simulink model "SPWM_Inverters"  (R2023a)
settings: Solver=ode23tb  StartTime=0.0  StopTime=1  MaxStep=1e-4  RelTol=1e-3
libraries: spsMosfetLib x22, spsSeriesRLCBranchLib x11, simulink x9, spsThreePhaseSeriesRLCBranchLib x8, spsDCVoltageSourceLib x7, spsVoltageMeasurementLib x7, spsThreePhaseVIMeasurementLib x6, spsGroundLib x3, spsPWMGenerator2LevelLib x2, spsUniversalBridgeLib x2, slpidlib x1, spsRMSLib x1
settings Model: Creator=gaming3  LastModifiedBy=gaming3

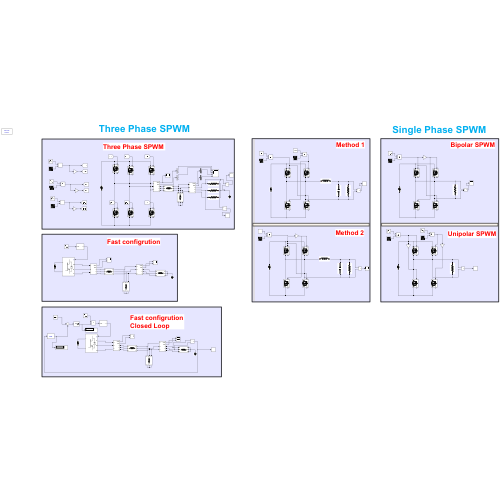
[thumbnail: Simulink's stored preview of the top-level diagram]
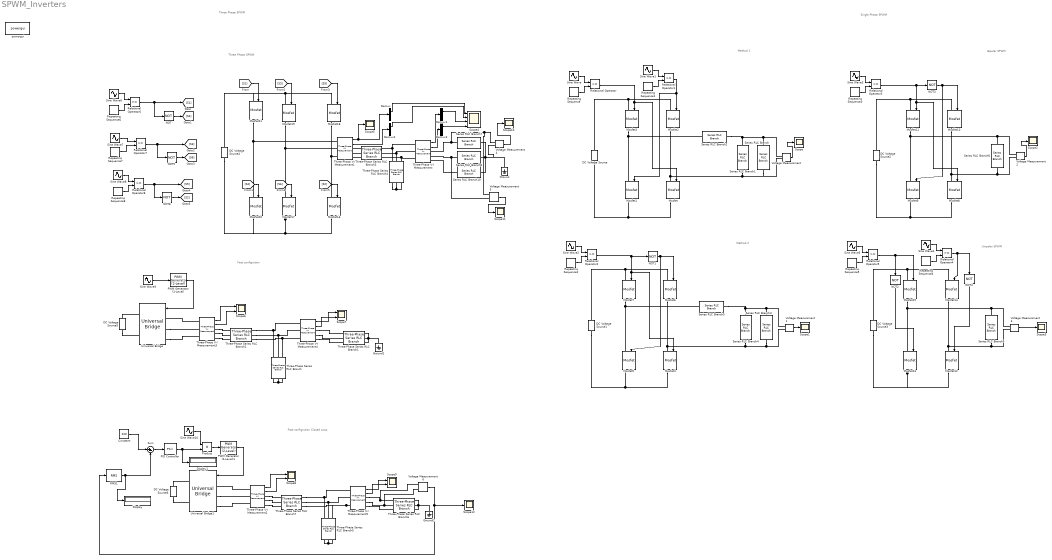
== system SPWM_Inverters ==
  note: Fast configrution
  note: Three Phase SPWM
  note: Bipolar SPWM
  note: Single Phase SPWM
  note: Unipolar SPWM
  note: Method 1
  note: Method 2
  note: Three Phase SPWM
  note: Fast configrution Closed Loop
  Constant : Constant  Value=220
  DC Voltage Source{,1..6} (7 alike) : spsDCVoltageSourceLib/DC Voltage Source  Amplitude=310  Measurements=None
  Demux{,1..3} (4 alike) : Demux  Outputs=3
  Display : Display
  Display1 : Display
  Ground : spsGroundLib/Ground  LConnTagsString=a
  Ground1 : spsGroundLib/Ground  LConnTagsString=a
  Ground2 : spsGroundLib/Ground  LConnTagsString=a
  Mosfet{,1..21} (22 alike) : spsMosfetLib/Mosfet  Ron=0.1  Lon=0  Rd=0.01  Vfd=0  IC=0  Rs=1e5  Cs=inf  Measurements=on
  NOT{,1..6} (7 alike) : Logic  Operator=NOT  IconShape=distinctive  AllPortsSameDT=off  OutDataTypeStr=boolean
  PID Controller : slpidlib/PID Controller  Controller=PI  Form=Parallel  TimeDomain=Continuous-time  UseExternalTs=off  SampleTime=-1  IntegratorMethod=Forward Euler  FilterMethod=Forward Euler  ControllerParametersSource=internal  P=0.0001  I=0.1  UseKiTs=off  D=0  N=100  UseFilter=on  TunerSelectOption=Transfer Function Based (PID Tuner App)  InitialConditionSource=internal  InitialConditionForIntegrator=0  InitialConditionForFilter=0  DifferentiatorICPrevScaledInput=0  ExternalReset=none  TrackingMode=off  Kt=1  LimitOutput=on  SatLimitsSource=internal  UpperSaturationLimit=0.98  LowerSaturationLimit=0  LinearizeAsGain=on  AntiWindupMode=none  Kb=1  LimitIntegrator=off  UpperIntegratorSaturationLimit=inf  LowerIntegratorSaturationLimit=-inf  POutMin=[]  POutMax=[]  IOutMin=[]  IOutMax=[]  DOutMin=[]  DOutMax=[]  NOutMin=[]  NOutMax=[]  SumOutMin=[]  SumOutMax=[]  SaturationOutMin=[]  SaturationOutMax=[]  PParamMin=[]  PParamMax=[]  IParamMin=[]  IParamMax=[]  DParamMin=[]  DParamMax=[]  NParamMin=[]  NParamMax=[]  KbParamMin=[]  KbParamMax=[]  KtParamMin=[]  KtParamMax=[]  KbOutMin=[]  KbOutMax=[]  KtOutMin=[]  KtOutMax=[]  IntegratorOutMin=[]  IntegratorOutMax=[]  FilterOutMin=[]  FilterOutMax=[]  SumI1OutMin=[]  SumI1OutMax=[]  SumI2OutMin=[]  SumI2OutMax=[]  SumI3OutMin=[]  SumI3OutMax=[]  SumI4OutMin=[]  SumI4OutMax=[]  SumDOutMin=[]  SumDOutMax=[]  DifferentiatorOutMin=[]  DifferentiatorOutMax=[]  FilterDiffOutCoefMin=[]  FilterDiffOutCoefMax=[]  ReciprocalOutMin=[]  ReciprocalOutMax=[]  SumDenOutMin=[]  SumDenOutMax=[]  SumNumOutMin=[]  SumNumOutMax=[]  DivideOutMin=[]  DivideOutMax=[]  UdiffTsProdOutMin=[]  UdiffTsProdOutMax=[]  NTsProdOutMin=[]  NTsProdOutMax=[]  UintegralTsProdOutMin=[]  UintegralTsProdOutMax=[]  UngainTsProdOutMin=[]  UngainTsProdOutMax=[]  ClampingZeroOutDataTypeStr=Inherit: Inherit via back propagation  ClampingZeroOutMin=[]  ClampingZeroOutMax=[]  FilterDenConstantOutDataTypeStr=Inherit: Inherit via back propagation  FilterDenConstantOutMin=[]  FilterDenConstantOutMax=[]  PCopyOutDataTypeStr=Inherit: Inherit via back propagation  PCopyOutMin=[]  PCopyOutMax=[]  NCopyOutDataTypeStr=Inherit: Inherit via back propagation  NCopyOutMin=[]  NCopyOutMax=[]  IntegratorContinuousStateAttributes=''  IntegratorStateMustResolveToSignalObject=off  IntegratorRTWStateStorageClass=Auto  FilterContinuousStateAttributes=''  FilterStateMustResolveToSignalObject=off  FilterRTWStateStorageClass=Auto  ParallelPVariant=InternalParameters  IdealPVariant=Disabled  IVariant=InternalParameters  DVariant=Disabled  IntegratorVariant=Continuous  SatVariant=Enabled  AWVariant=Passthrough  PCopyVariant=Disabled  TRVariant=Disabled  FdbkBlocksVariant=Forward  IdealPFdbkVariant=Disabled  SatFdbkVariant=Disabled  DerivativeFilterVariant=Disabled  NVariant=Disabled  NCopyVariant=Disabled_SignalSpec  FilterICVariant=Disabled  IntegratorICVariant=InternalICs  ExternalResetVariant=Disabled  TRSumVariant=Passthrough  SumFdbkVariant=Disabled  SumVariant=Sum_PI  TsampFilterVariant=InternalTs  TsampNgainVariant=Passthrough  TsampIntegralVariant=Disabled_SignalSpec  ExternalSaturationOutDataTypeStr=Inherit: Same as second input
  PWM Generator (2-Level) : spsPWMGenerator2LevelLib/PWM Generator (2-Level)  ModulatorType=Three-phase bridge (6 pulses)  ModulatorMode=Unsynchronized  Fc=101*50  Pc=90  nF=27  MinMax="[ -1  1 ]"  SamplingTechnique=Natural  ModulatingSignals=off  m=0.8  Freq=60  Phase=0  Ts=0  ShowCarrierOutport=off
  PWM Generator (2-Level)1 : spsPWMGenerator2LevelLib/PWM Generator (2-Level)  ModulatorType=Three-phase bridge (6 pulses)  ModulatorMode=Unsynchronized  Fc=101*50  Pc=90  nF=27  MinMax="[ -1  1 ]"  SamplingTechnique=Natural  ModulatingSignals=off  m=0.8  Freq=60  Phase=0  Ts=0  ShowCarrierOutport=off
  Product : Product
  RMS1 : spsRMSLib/RMS  TrueRMS=on  Freq=50  RMSInit=0  Ts=0
  Relational Operator{,1..8} (9 alike) : RelationalOperator  OutDataTypeStr=boolean  RndMeth=Simplest  InputSameDT=off
  Repeating Sequence{,1..5} (6 alike) : simulink/Sources/Repeating Sequence  rep_seq_t=[0 (1/5000)/4 (1/5000)/2 (3/5000)/4 (1/5000)]  rep_seq_y=[0 1 0 -1 0]
  Repeating Sequence6 : simulink/Sources/Repeating Sequence  rep_seq_t=[0 (0.25/5000) (0.5/5000) (0.75/5000) (1/5000)]  rep_seq_y=[0 1 0 -1 0]
  Repeating Sequence7 : simulink/Sources/Repeating Sequence  rep_seq_t=[0 (0.25/5000) (0.5/5000) (0.75/5000) (1/5000)]  rep_seq_y=[0 1 0 -1 0]
  Repeating Sequence8 : simulink/Sources/Repeating Sequence  rep_seq_t=[0 (0.25/5000) (0.5/5000) (0.75/5000) (1/5000)]  rep_seq_y=[0 1 0 -1 0]
  Scope{,1..3,5,10..12} (8 alike) : Scope
  Scope4 : Scope  NumInputPorts=4
  Scope{6..9} (4 alike) : Scope  NumInputPorts=2
  Series RLC Branch{,3,6,9} (4 alike) : spsSeriesRLCBranchLib/Series RLC Branch  LConnTagsString=__new0  RConnTagsString=__new0  BranchType=R  Resistance=100  Inductance=1e-3  SetiL0=off  InitialCurrent=0  Capacitance=1e-6  Setx0=off  InitialVoltage=0  Measurements=None
  Series RLC Branch1 : spsSeriesRLCBranchLib/Series RLC Branch  LConnTagsString=__new0  RConnTagsString=__new0  BranchType=C  Resistance=100  Inductance=1e-3  SetiL0=off  InitialCurrent=0  Capacitance=1000e-6  Setx0=off  InitialVoltage=0  Measurements=None
  Series RLC Branch10 : spsSeriesRLCBranchLib/Series RLC Branch  LConnTagsString=__new0  RConnTagsString=__new0  BranchType=R  Resistance=10  Inductance=1e-3  SetiL0=off  InitialCurrent=0  Capacitance=1e-6  Setx0=off  InitialVoltage=0  Measurements=None
  Series RLC Branch2 : spsSeriesRLCBranchLib/Series RLC Branch  LConnTagsString=__new0  RConnTagsString=__new0  BranchType=L  Resistance=100  Inductance=0.00001  SetiL0=off  InitialCurrent=0  Capacitance=1e-6  Setx0=off  InitialVoltage=0  Measurements=None
  Series RLC Branch4 : spsSeriesRLCBranchLib/Series RLC Branch  LConnTagsString=__new0  RConnTagsString=__new0  BranchType=C  Resistance=100  Inductance=1e-3  SetiL0=off  InitialCurrent=0  Capacitance=500e-6  Setx0=off  InitialVoltage=0  Measurements=None
  Series RLC Branch5 : spsSeriesRLCBranchLib/Series RLC Branch  LConnTagsString=__new0  RConnTagsString=__new0  BranchType=L  Resistance=100  Inductance=0.001  SetiL0=off  InitialCurrent=0  Capacitance=1e-6  Setx0=off  InitialVoltage=0  Measurements=None
  Series RLC Branch7 : spsSeriesRLCBranchLib/Series RLC Branch  LConnTagsString=__new0  RConnTagsString=__new0  BranchType=R  Resistance=10  Inductance=1e-3  SetiL0=off  InitialCurrent=0  Capacitance=1e-6  Setx0=off  InitialVoltage=0  Measurements=None
  Series RLC Branch8 : spsSeriesRLCBranchLib/Series RLC Branch  LConnTagsString=__new0  RConnTagsString=__new0  BranchType=R  Resistance=10  Inductance=1e-3  SetiL0=off  InitialCurrent=0  Capacitance=1e-6  Setx0=off  InitialVoltage=0  Measurements=None
  Sine Wave{,2..3,5} (4 alike) : Sin  Amplitude=0.95  Frequency=100*pi  SampleTime=0
  Sine Wave1 : Sin  Amplitude=0.95  Frequency=100*pi  Phase=pi  SampleTime=0
  Sine Wave10 : Sin  Frequency=100*pi  Phase="[0 -(2*pi)/3  (2*pi)/3 ]"  SampleTime=0
  Sine Wave4 : Sin  Amplitude=0.95  Frequency=100*pi  Phase=pi  SampleTime=0
  Sine Wave6 : Sin  Amplitude=.99  Frequency=100*pi  SampleTime=0
  Sine Wave7 : Sin  Amplitude=0.99  Frequency=100*pi  Phase=(2*pi)/3  SampleTime=0
  Sine Wave8 : Sin  Amplitude=0.99  Frequency=100*pi  Phase=(4*pi)/3  SampleTime=0
  Sine Wave9 : Sin  Amplitude=0.99  Frequency=100*pi  Phase="[0 -(2*pi)/3  (2*pi)/3 ]"  SampleTime=0
  Sum : Sum  Inputs=|+-
  Three-Phase Series RLC Branch : spsThreePhaseSeriesRLCBranchLib/Three-Phase Series RLC Branch  LConnTagsString=A|B|C  RConnTagsString=A|B|C  BranchType=C  Resistance=1  Inductance=1e-3  Capacitance=500e-6  Measurements=None
  Three-Phase Series RLC Branch1 : spsThreePhaseSeriesRLCBranchLib/Three-Phase Series RLC Branch  LConnTagsString=A|B|C  RConnTagsString=A|B|C  BranchType=R  Resistance=10  Inductance=1e-3  Capacitance=1e-6  Measurements=None
  Three-Phase Series RLC Branch2 : spsThreePhaseSeriesRLCBranchLib/Three-Phase Series RLC Branch  LConnTagsString=A|B|C  RConnTagsString=A|B|C  BranchType=L  Resistance=1  Inductance=5e-3  Capacitance=1e-6  Measurements=None
  Three-Phase Series RLC Branch3 : spsThreePhaseSeriesRLCBranchLib/Three-Phase Series RLC Branch  LConnTagsString=A|B|C  RConnTagsString=A|B|C  BranchType=L  Resistance=1  Inductance=5e-3  Capacitance=1e-6  Measurements=None
  Three-Phase Series RLC Branch4 : spsThreePhaseSeriesRLCBranchLib/Three-Phase Series RLC Branch  LConnTagsString=A|B|C  RConnTagsString=A|B|C  BranchType=C  Resistance=1  Inductance=1e-3  Capacitance=500e-6  Measurements=None
  Three-Phase Series RLC Branch5 : spsThreePhaseSeriesRLCBranchLib/Three-Phase Series RLC Branch  LConnTagsString=A|B|C  RConnTagsString=A|B|C  BranchType=C  Resistance=1  Inductance=1e-3  Capacitance=500e-6  Measurements=None
  Three-Phase Series RLC Branch6 : spsThreePhaseSeriesRLCBranchLib/Three-Phase Series RLC Branch  LConnTagsString=A|B|C  RConnTagsString=A|B|C  BranchType=R  Resistance=10  Inductance=1e-3  Capacitance=1e-6  Measurements=None
  Three-Phase Series RLC Branch7 : spsThreePhaseSeriesRLCBranchLib/Three-Phase Series RLC Branch  LConnTagsString=A|B|C  RConnTagsString=A|B|C  BranchType=L  Resistance=1  Inductance=5e-3  Capacitance=1e-6  Measurements=None
  Three-Phase V-I Measurement : spsThreePhaseVIMeasurementLib/Three-Phase V-I Measurement  VoltageMeasurement=phase-to-phase  SetLabelV=off  LabelV=Vabc  Vpu=off  VpuLL=off  CurrentMeasurement=yes  SetLabelI=off  LabelI=Iabc  Ipu=off  Pbase=100e6  Vbase=500e3  OutputType=Complex  PhasorSimulation=off  PSBequivalent=0
  Three-Phase V-I Measurement1 : spsThreePhaseVIMeasurementLib/Three-Phase V-I Measurement  VoltageMeasurement=phase-to-ground  SetLabelV=off  LabelV=Vabc  Vpu=off  VpuLL=off  CurrentMeasurement=yes  SetLabelI=off  LabelI=Iabc  Ipu=off  Pbase=100e6  Vbase=500e3  OutputType=Complex  PhasorSimulation=off  PSBequivalent=0
  Three-Phase V-I Measurement2 : spsThreePhaseVIMeasurementLib/Three-Phase V-I Measurement  VoltageMeasurement=phase-to-phase  SetLabelV=off  LabelV=Vabc  Vpu=off  VpuLL=off  CurrentMeasurement=yes  SetLabelI=off  LabelI=Iabc  Ipu=off  Pbase=100e6  Vbase=500e3  OutputType=Complex  PhasorSimulation=off  PSBequivalent=0
  Three-Phase V-I Measurement3 : spsThreePhaseVIMeasurementLib/Three-Phase V-I Measurement  VoltageMeasurement=phase-to-phase  SetLabelV=off  LabelV=Vabc  Vpu=off  VpuLL=off  CurrentMeasurement=yes  SetLabelI=off  LabelI=Iabc  Ipu=off  Pbase=100e6  Vbase=500e3  OutputType=Complex  PhasorSimulation=off  PSBequivalent=0
  Three-Phase V-I Measurement4 : spsThreePhaseVIMeasurementLib/Three-Phase V-I Measurement  VoltageMeasurement=phase-to-ground  SetLabelV=off  LabelV=Vabc  Vpu=off  VpuLL=off  CurrentMeasurement=yes  SetLabelI=off  LabelI=Iabc  Ipu=off  Pbase=100e6  Vbase=500e3  OutputType=Complex  PhasorSimulation=off  PSBequivalent=0
  Three-Phase V-I Measurement5 : spsThreePhaseVIMeasurementLib/Three-Phase V-I Measurement  VoltageMeasurement=phase-to-ground  SetLabelV=off  LabelV=Vabc  Vpu=off  VpuLL=off  CurrentMeasurement=yes  SetLabelI=off  LabelI=Iabc  Ipu=off  Pbase=100e6  Vbase=500e3  OutputType=Complex  PhasorSimulation=off  PSBequivalent=0
  Universal Bridge : spsUniversalBridgeLib/Universal Bridge  Arms=3  SnubberResistance=1e5  SnubberCapacitance=inf  Device=IGBT / Diodes  Ron=1e-3  Lon=0  ForwardVoltages="[  0  0  ]"  ForwardVoltage=0  GTOparameters=[ 10e-6 , 20e-6 ]  IGBTparameters=[ 1e-6 , 2e-6 ]  Measurements=None  Measurements_2=None  converterType=Rectifier
  Universal Bridge1 : spsUniversalBridgeLib/Universal Bridge  Arms=3  SnubberResistance=1e5  SnubberCapacitance=inf  Device=IGBT / Diodes  Ron=1e-3  Lon=0  ForwardVoltages="[  0  0  ]"  ForwardVoltage=0  GTOparameters=[ 10e-6 , 20e-6 ]  IGBTparameters=[ 1e-6 , 2e-6 ]  Measurements=None  Measurements_2=None  converterType=Rectifier
  Voltage Measurement{,1..6} (7 alike) : spsVoltageMeasurementLib/Voltage Measurement  PhasorSimulation=off  OutputType=Complex  PSBequivalent=0
  powergui : spspowerguiLib/powergui  Priority=1  SimulationMode=Discrete  SampleTime=1e-06  frequency=60  Iterations=50  frequencyindice=0  Pbase=100e6  ErrMax=1e-4  UnitsV=kV  UnitsW=MW  buscounter=0  FunctionMessages=off  echomessages=off  EnableUseOfTLC=off  CurrentSourceSwitches=off  DisableSnubberDevices=off  DisableRonSwitches=off  DisableVfSwitches=off  DisplayEquations=off  AutomaticDiscreteSolvers=off  SolverType=Tustin/Backward Euler (TBE)  Interpol=off  ExternalGateDelay=off  methode=off  Ts=100  x0status=blocks  SPID=on  SwTol=0  HookPort=off  NonlinearTolerance=1e-4  nMaxIteration=100  ContinueOnMaxIteration=off  RestoreLinks=warning  ResistiveCurrentMeasurement=off  Frange=[0:2:500]  Ylog=off  Xlog=on  ShowGrid=off  save=off  variable=ZData  structure=0  ZoomFFT=off  StartTime=0.0  cycles=1  DisplayStyle=1  fundamental=60  FreqAxis=off  MaxFrequency=1000  frequencyindicesteady=1  RmsSteady=1  display=off
  wires:
  Voltage Measurement/1 -> Scope/1
  Sine Wave/1 -> Relational Operator/1
  Repeating Sequence/1 -> Relational Operator/2
  Relational Operator/1 -> Mosfet/1, Mosfet3/1
  Repeating Sequence1/1 -> Relational Operator1/2
  Sine Wave1/1 -> Relational Operator1/1
  Relational Operator1/1 -> Mosfet1/1, Mosfet2/1
  Relational Operator2/1 -> NOT1/1, Mosfet7/1, Mosfet4/1
  Repeating Sequence2/1 -> Relational Operator2/2
  Sine Wave2/1 -> Relational Operator2/1
  Voltage Measurement1/1 -> Scope1/1
  NOT1/1 -> Mosfet6/1, Mosfet5/1
  Voltage Measurement3/1 -> Scope3/1
  Sine Wave5/1 -> Relational Operator5/1
  Repeating Sequence5/1 -> Relational Operator5/2
  Relational Operator5/1 -> Mosfet15/1, NOT2/1
  Relational Operator3/1 -> NOT3/1, Mosfet11/1, Mosfet8/1
  Repeating Sequence3/1 -> Relational Operator3/2
  Sine Wave3/1 -> Relational Operator3/1
  Voltage Measurement2/1 -> Scope2/1
  NOT3/1 -> Mosfet10/1, Mosfet9/1
  NOT2/1 -> Mosfet13/1
  Relational Operator4/1 -> NOT4/1, Mosfet14/1
  Repeating Sequence4/1 -> Relational Operator4/2
  Sine Wave4/1 -> Relational Operator4/1
  NOT4/1 -> Mosfet12/1
  [S6] -> Mosfet17/1
  NOT6/1 -> [S2]
  Three-Phase V-I Measurement/1 -> Demux1/1
  [S5] -> Mosfet18/1
  Three-Phase V-I Measurement1/1 -> Demux/1, Scope5/1
  [S1] -> Mosfet21/1
  Demux1/1 -> Scope4/3
  Demux/1 -> Scope4/1
  [S4] -> Mosfet20/1
  Demux3/1 -> Scope4/4
  Relational Operator7/1 -> [S3], NOT5/1
  Demux2/1 -> Scope4/2
  NOT5/1 -> [S6]
  NOT/1 -> [S4]
  Three-Phase V-I Measurement1/2 -> Demux2/1
  [S3] -> Mosfet19/1
  [S2] -> Mosfet16/1
  Three-Phase V-I Measurement/2 -> Demux3/1
  Repeating Sequence6/1 -> Relational Operator6/2
  Sine Wave6/1 -> Relational Operator6/1
  Relational Operator6/1 -> NOT/1, [S1]
  Repeating Sequence7/1 -> Relational Operator7/2
  Sine Wave8/1 -> Relational Operator8/1
  Repeating Sequence8/1 -> Relational Operator8/2
  Relational Operator8/1 -> NOT6/1, [S5]
  Sine Wave7/1 -> Relational Operator7/1
  Sine Wave9/1 -> PWM Generator (2-Level)/1
  PWM Generator (2-Level)/1 -> Universal Bridge/1
  Three-Phase V-I Measurement3/1 -> Scope6/1
  Three-Phase V-I Measurement3/2 -> Scope6/2
  Three-Phase V-I Measurement4/1 -> Scope7/1
  Three-Phase V-I Measurement4/2 -> Scope7/2
  Three-Phase V-I Measurement5/2 -> Scope9/2
  Three-Phase V-I Measurement5/1 -> Scope9/1
  Three-Phase V-I Measurement2/2 -> Scope8/2
  Three-Phase V-I Measurement2/1 -> Scope8/1
  PWM Generator (2-Level)1/1 -> Universal Bridge1/1
  Voltage Measurement4/1 -> Scope10/1
  Voltage Measurement5/1 -> Scope11/1
  Product/1 -> PWM Generator (2-Level)1/1
  Sine Wave10/1 -> Product/1
  RMS1/1 -> Display/1, Sum/2
  Constant/1 -> Sum/1
  Sum/1 -> PID Controller/1
  PID Controller/1 -> Display1/1, Product/2
  Voltage Measurement6/1 -> Scope12/1, RMS1/1
  connections:
  Mosfet3/LConn1 -- DC Voltage Source/RConn1 -- Mosfet2/LConn1
  Voltage Measurement/LConn1 -- Series RLC Branch/LConn1 -- Series RLC Branch1/LConn1 -- Series RLC Branch2/RConn1
  Mosfet2/RConn1 -- Series RLC Branch/RConn1 -- Voltage Measurement/LConn2 -- Series RLC Branch1/RConn1 -- Mosfet/LConn1
  Mosfet/RConn1 -- DC Voltage Source/LConn1 -- Mosfet1/RConn1
  Mosfet3/RConn1 -- Series RLC Branch2/LConn1 -- Mosfet1/LConn1
  DC Voltage Source1/RConn1 -- Mosfet7/LConn1 -- Mosfet6/LConn1
  Series RLC Branch3/LConn1 -- Voltage Measurement1/LConn1 -- Series RLC Branch5/RConn1 -- Series RLC Branch4/LConn1
  Series RLC Branch3/RConn1 -- Voltage Measurement1/LConn2 -- Series RLC Branch4/RConn1 -- Mosfet4/LConn1 -- Mosfet6/RConn1
  Mosfet4/RConn1 -- Mosfet5/RConn1 -- DC Voltage Source1/LConn1
  Series RLC Branch5/LConn1 -- Mosfet7/RConn1 -- Mosfet5/LConn1
  DC Voltage Source2/RConn1 -- Mosfet11/LConn1 -- Mosfet10/LConn1
  Series RLC Branch6/RConn1 -- Voltage Measurement2/LConn2 -- Mosfet8/LConn1 -- Mosfet10/RConn1
  Mosfet8/RConn1 -- Mosfet9/RConn1 -- DC Voltage Source2/LConn1
  Series RLC Branch6/LConn1 -- Mosfet9/LConn1 -- Mosfet11/RConn1 -- Voltage Measurement2/LConn1
  Mosfet15/LConn1 -- DC Voltage Source3/RConn1 -- Mosfet14/LConn1
  Voltage Measurement3/LConn2 -- Mosfet14/RConn1 -- Mosfet12/LConn1 -- Series RLC Branch9/RConn1
  Mosfet13/RConn1 -- Mosfet12/RConn1 -- DC Voltage Source3/LConn1
  Voltage Measurement3/LConn1 -- Mosfet15/RConn1 -- Mosfet13/LConn1 -- Series RLC Branch9/LConn1
  Mosfet19/RConn1 -- Three-Phase V-I Measurement1/LConn2 -- Mosfet17/LConn1
  Mosfet19/LConn1 -- DC Voltage Source4/RConn1 -- Mosfet21/LConn1 -- Mosfet18/LConn1
  Mosfet17/RConn1 -- Mosfet16/RConn1 -- Mosfet20/RConn1 -- DC Voltage Source4/LConn1
  Mosfet21/RConn1 -- Mosfet20/LConn1 -- Three-Phase V-I Measurement1/LConn1
  Mosfet18/RConn1 -- Three-Phase V-I Measurement1/LConn3 -- Mosfet16/LConn1
  Series RLC Branch7/LConn1 -- Voltage Measurement4/LConn2 -- Ground/LConn1 -- Series RLC Branch8/LConn1 -- Series RLC Branch10/LConn1
  Series RLC Branch8/RConn1 -- Voltage Measurement5/LConn2 -- Three-Phase V-I Measurement/RConn2
  Series RLC Branch7/RConn1 -- Voltage Measurement5/LConn1 -- Voltage Measurement4/LConn1 -- Three-Phase V-I Measurement/RConn1
  Series RLC Branch10/RConn1 -- Three-Phase V-I Measurement/RConn3
  DC Voltage Source5/RConn1 -- Universal Bridge/RConn1
  DC Voltage Source5/LConn1 -- Universal Bridge/RConn2
  Three-Phase V-I Measurement3/LConn1 -- Universal Bridge/LConn1
  Universal Bridge/LConn2 -- Three-Phase V-I Measurement3/LConn2
  Universal Bridge/LConn3 -- Three-Phase V-I Measurement3/LConn3
  Three-Phase V-I Measurement4/RConn1 -- Three-Phase Series RLC Branch1/LConn1
  Three-Phase V-I Measurement4/RConn2 -- Three-Phase Series RLC Branch1/LConn2
  Three-Phase V-I Measurement4/RConn3 -- Three-Phase Series RLC Branch1/LConn3
  Three-Phase Series RLC Branch1/RConn1 -- Ground1/LConn1 -- Three-Phase Series RLC Branch1/RConn2 -- Three-Phase Series RLC Branch1/RConn3
  Three-Phase V-I Measurement3/RConn1 -- Three-Phase Series RLC Branch2/LConn1
  Three-Phase V-I Measurement3/RConn2 -- Three-Phase Series RLC Branch2/LConn2
  Three-Phase V-I Measurement3/RConn3 -- Three-Phase Series RLC Branch2/LConn3
  Three-Phase Series RLC Branch2/RConn1 -- Three-Phase Series RLC Branch/LConn1 -- Three-Phase V-I Measurement4/LConn1
  Three-Phase Series RLC Branch2/RConn2 -- Three-Phase Series RLC Branch/LConn2 -- Three-Phase V-I Measurement4/LConn2
  Three-Phase Series RLC Branch2/RConn3 -- Three-Phase V-I Measurement4/LConn3 -- Three-Phase Series RLC Branch/LConn3
  Three-Phase Series RLC Branch/RConn1 -- Three-Phase Series RLC Branch/RConn2 -- Three-Phase Series RLC Branch/RConn3
  Three-Phase Series RLC Branch4/RConn1 -- Three-Phase Series RLC Branch4/RConn2 -- Three-Phase Series RLC Branch4/RConn3
  Three-Phase Series RLC Branch3/LConn1 -- Three-Phase V-I Measurement1/RConn1
  Three-Phase Series RLC Branch3/LConn2 -- Three-Phase V-I Measurement1/RConn2
  Three-Phase Series RLC Branch3/LConn3 -- Three-Phase V-I Measurement1/RConn3
  Three-Phase Series RLC Branch4/LConn1 -- Three-Phase V-I Measurement/LConn1 -- Three-Phase Series RLC Branch3/RConn1
  Three-Phase Series RLC Branch4/LConn2 -- Three-Phase V-I Measurement/LConn2 -- Three-Phase Series RLC Branch3/RConn2
  Three-Phase Series RLC Branch4/LConn3 -- Three-Phase V-I Measurement/LConn3 -- Three-Phase Series RLC Branch3/RConn3
  Ground2/LConn1 -- Three-Phase Series RLC Branch6/RConn1 -- Three-Phase Series RLC Branch6/RConn3 -- Three-Phase Series RLC Branch6/RConn2
  Three-Phase Series RLC Branch5/LConn1 -- Three-Phase Series RLC Branch7/RConn1 -- Three-Phase V-I Measurement5/LConn1
  Three-Phase Series RLC Branch5/LConn2 -- Three-Phase Series RLC Branch7/RConn2 -- Three-Phase V-I Measurement5/LConn2
  Three-Phase V-I Measurement5/LConn3 -- Three-Phase Series RLC Branch7/RConn3 -- Three-Phase Series RLC Branch5/LConn3
  Three-Phase Series RLC Branch5/RConn2 -- Three-Phase Series RLC Branch5/RConn1 -- Three-Phase Series RLC Branch5/RConn3
  Three-Phase V-I Measurement2/RConn3 -- Three-Phase Series RLC Branch7/LConn3
  Three-Phase V-I Measurement2/RConn2 -- Three-Phase Series RLC Branch7/LConn2
  Three-Phase V-I Measurement2/RConn1 -- Three-Phase Series RLC Branch7/LConn1
  Universal Bridge1/LConn3 -- Three-Phase V-I Measurement2/LConn3
  Three-Phase V-I Measurement5/RConn2 -- Voltage Measurement6/LConn2 -- Three-Phase Series RLC Branch6/LConn2
  Universal Bridge1/LConn2 -- Three-Phase V-I Measurement2/LConn2
  Three-Phase V-I Measurement5/RConn3 -- Three-Phase Series RLC Branch6/LConn3
  Three-Phase V-I Measurement2/LConn1 -- Universal Bridge1/LConn1
  DC Voltage Source6/LConn1 -- Universal Bridge1/RConn2
  DC Voltage Source6/RConn1 -- Universal Bridge1/RConn1
  Three-Phase V-I Measurement5/RConn1 -- Voltage Measurement6/LConn1 -- Three-Phase Series RLC Branch6/LConn1
